simulink model "SimulinkMotor"  (R2019a)
settings: Solver=VariableStepAuto  StartTime=0.0  StopTime=20  RelTol=1e-3
libraries: fuzblock x1
settings Model: Creator=user  LastModifiedBy=user

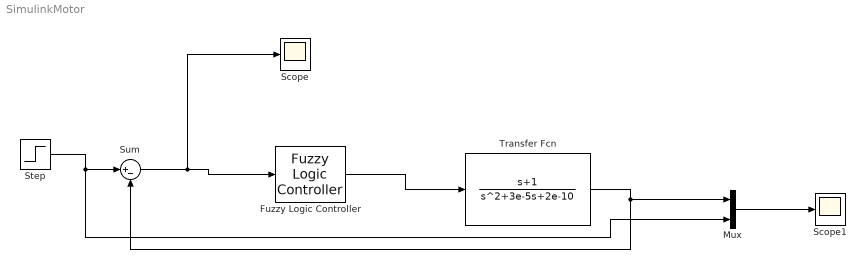
== system SimulinkMotor ==
  Fuzzy Logic Controller : fuzblock/Fuzzy Logic  Controller  FIS='Motor2.fis'  OutputSampleNumber=101  DataType=double  FuzzifiedInputs=off  RuleFiringStrengths=off  RuleOutputs=off  AggregatedOutputs=off  SimulateUsing=Interpreted execution  OutOfRangeInputValueMessage=warning  NoRuleFiredMessage=warning  EmptyOutputFuzzySetMessage=warning
  Mux : Mux  Inputs=2
  Scope : Scope
  Scope1 : Scope
  Step : Step  Time=20  SampleTime=0
  Sum : Sum  Inputs=|+-
  Transfer Fcn : TransferFcn  Numerator=[1 1]  Denominator=[1 3e-5 2e-10]
  wires:
  Transfer Fcn/1 -> Mux/1, Sum/2
  Sum/1 -> Scope/1, Fuzzy Logic Controller/1
  Fuzzy Logic Controller/1 -> Transfer Fcn/1
  Mux/1 -> Scope1/1
  Step/1 -> Mux/2, Sum/1
